simulink model "CRA_Assignment2"  (R2022b)
settings: Solver=ode23  StartTime=0.0  StopTime=10  RelTol=1e-7  AbsTol=1e-7
libraries: simulink x2
settings Model: Creator=gianm  LastModifiedBy=lerio

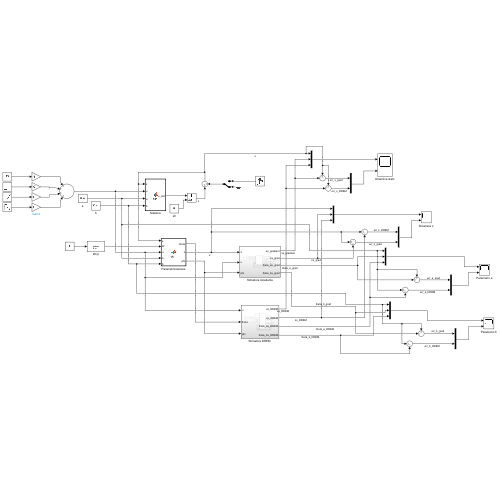
[thumbnail: Simulink's stored preview of the top-level diagram]
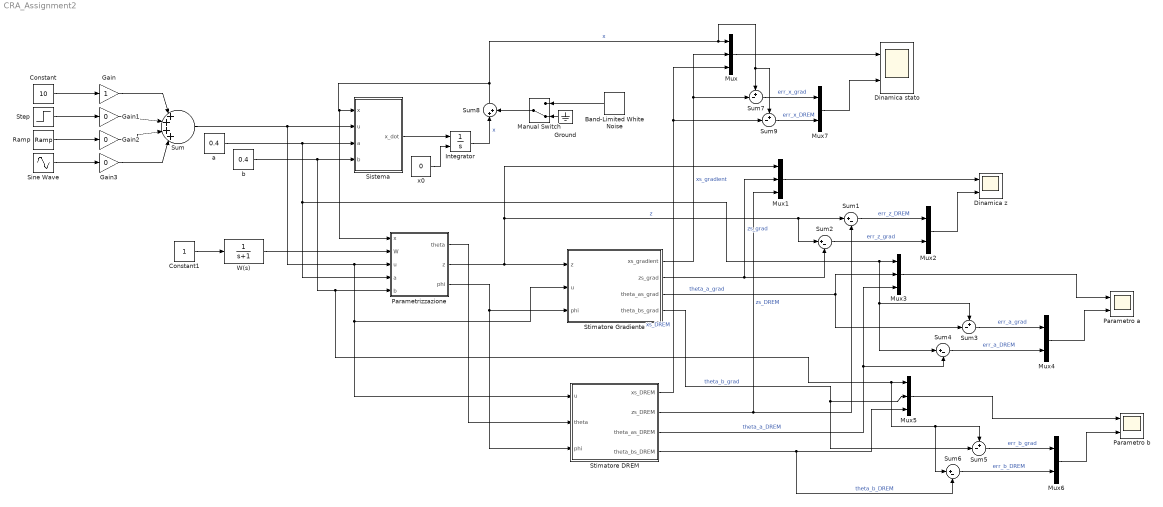
== system CRA_Assignment2 ==
  Band-Limited White Noise : simulink/Sources/Band-Limited White Noise  Cov=[0.02]  Ts=0.1  seed=[23341]
  Constant : Constant  Value=10
  Constant1 : Constant
  Dinamica stato : Scope  NumInputPorts=2
  Dinamica z : Scope  NumInputPorts=2
  Gain : Gain
  Gain1 : Gain  Gain=0
  Gain2 : Gain  Gain=0
  Gain3 : Gain  Gain=0
  Ground : Ground
  Integrator : Integrator  InitialConditionSource=external
  Manual Switch : ManualSwitch  CurrentSetting=0
  Mux{,1,3,5} (4 alike) : Mux  Inputs=3
  Mux{2,4,6..7} (4 alike) : Mux  Inputs=2
  Parametrizzazione : MATLAB Function  TreatAsAtomicUnit=on
  Parametro a : Scope  NumInputPorts=2
  Parametro b : Scope  NumInputPorts=2
  Ramp : simulink/Sources/Ramp  slope=1  start=0  InitialOutput=0
  Sine Wave : Sin  Amplitude=10  Frequency=5/2  SampleTime=0
  Sistema : MATLAB Function  TreatAsAtomicUnit=on
  Step : Step  After=10  SampleTime=0
  "Stimatore DREM " : Subsystem
  Stimatore Gradiente : Subsystem
  Sum : Sum  Inputs=|++++|
  Sum{1..2,4,6} (4 alike) : Sum  Inputs=|+-
  Sum{3,5,7,9} (4 alike) : Sum  Inputs=+-|
  Sum8 : Sum  Inputs=|++
  W(s) : TransferFcn  Denominator=[1 1]
  a : Constant  Value=0.4
  b : Constant  Value=0.4
  x0 : Constant  Value=0
  wires:
  Sistema/1(x_dot) -> Integrator/1
  Gain/1 -> Sum/1
  Gain1/1 -> Sum/2
  Gain2/1 -> Sum/3
  Gain3/1 -> Sum/4
  Sum/1 -> "Stimatore DREM "/1(u), Stimatore Gradiente/2(u), Parametrizzazione/3(u), Sistema/2(u)
  Constant/1 -> Gain/1
  Step/1 -> Gain1/1
  Ramp/1 -> Gain2/1
  Sine Wave/1 -> Gain3/1
  b/1 -> Sum6/1, Sum5/1, Mux5/1, Parametrizzazione/5(b), Sistema/4(b)
  a/1 -> Sum3/1, Sum4/1, Mux3/1, Parametrizzazione/4(a), Sistema/3(a)
  Constant1/1 -> W(s)/1
  W(s)/1 -> Parametrizzazione/2(W)
  Parametrizzazione/3(phi) -> "Stimatore DREM "/3(phi), Stimatore Gradiente/3(phi)
  Parametrizzazione/2(z) -> Sum2/1, Sum1/1, Mux1/1, Stimatore Gradiente/1(z)  "z"
  Parametrizzazione/1(theta) -> "Stimatore DREM "/2(theta)
  x0/1 -> Integrator/2
  Mux/1 -> Dinamica stato/1
  Stimatore Gradiente/1(xs_gradient) -> Sum7/2, Mux/2  "xs_gradient"
  "Stimatore DREM "/1(xs_DREM) -> Sum9/2, Mux/3  "xs_DREM"
  Stimatore Gradiente/2(zs_grad) -> Sum2/2, Mux1/2  "zs_grad"
  "Stimatore DREM "/2(zs_DREM) -> Sum1/2, Mux1/3  "zs_DREM"
  Mux1/1 -> Dinamica z/1
  Sum1/1 -> Mux2/1  "err_z_DREM"
  Sum2/1 -> Mux2/2  "err_z_grad"
  Mux2/1 -> Dinamica z/2
  Mux3/1 -> Parametro a/1
  Sum4/1 -> Mux4/2  "err_a_DREM"
  Mux4/1 -> Parametro a/2
  Sum3/1 -> Mux4/1  "err_a_grad"
  Stimatore Gradiente/3(theta_as_grad) -> Sum3/2, Mux3/2  "theta_a_grad"
  "Stimatore DREM "/3(theta_as_DREM) -> Sum4/2, Mux3/3  "theta_a_DREM"
  Mux6/1 -> Parametro b/2
  Sum5/1 -> Mux6/1  "err_b_grad"
  Sum6/1 -> Mux6/2  "err_b_DREM"
  Mux5/1 -> Parametro b/1
  "Stimatore DREM "/4(theta_bs_DREM) -> Mux5/3, Sum6/2  "theta_b_DREM"
  Stimatore Gradiente/4(theta_bs_grad) -> Sum5/2, Mux5/2  "theta_b_grad"
  Sum9/1 -> Mux7/2  "err_x_DREM"
  Sum7/1 -> Mux7/1  "err_x_grad"
  Mux7/1 -> Dinamica stato/2
  Integrator/1 -> Sum8/1  "x"
  Manual Switch/1 -> Sum8/2
  Ground/1 -> Manual Switch/2
  Band-Limited White Noise/1 -> Manual Switch/1
  Sum8/1 -> Sum9/1, Sum7/1, Mux/1, Parametrizzazione/1(x), Sistema/1(x)  "x"

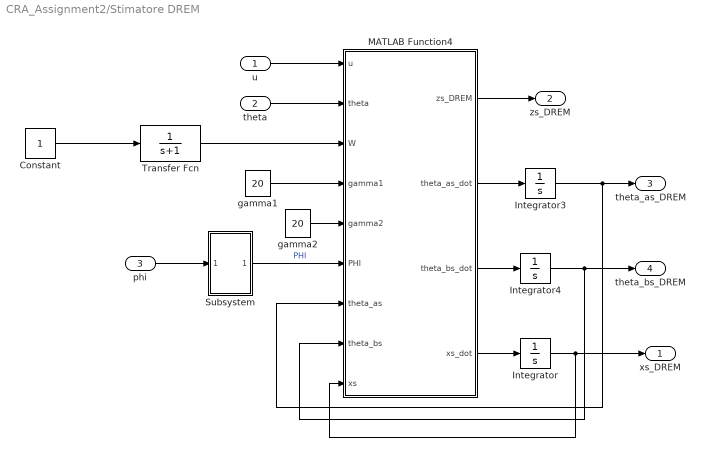
== system CRA_Assignment2/Stimatore DREM  ==
  u : Inport
  theta : Inport  Port=2
  phi : Inport  Port=3
  Constant : Constant
  Integrator : Integrator
  Integrator3 : Integrator
  Integrator4 : Integrator
  MATLAB Function4 : MATLAB Function  TreatAsAtomicUnit=on
  Subsystem : Subsystem
  Transfer Fcn : TransferFcn  Denominator=[1 1]
  gamma1 : Constant  Value=20
  gamma2 : Constant  Value=20
  xs_DREM : Outport
  zs_DREM : Outport  Port=2
  theta_as_DREM : Outport  Port=3
  theta_bs_DREM : Outport  Port=4
  wires:
  MATLAB Function4/2(theta_as_dot) -> Integrator3/1
  theta/1 -> MATLAB Function4/2(theta)
  gamma1/1 -> MATLAB Function4/4(gamma1)
  phi/1 -> Subsystem/1(phi)
  Integrator4/1 -> theta_bs_DREM/1, MATLAB Function4/8(theta_bs)
  gamma2/1 -> MATLAB Function4/5(gamma2)
  MATLAB Function4/1(zs_DREM) -> zs_DREM/1
  MATLAB Function4/3(theta_bs_dot) -> Integrator4/1
  Integrator3/1 -> MATLAB Function4/7(theta_as), theta_as_DREM/1
  Subsystem/1(PHI) -> MATLAB Function4/6(PHI)  "PHI"
  MATLAB Function4/4(xs_dot) -> Integrator/1
  Integrator/1 -> MATLAB Function4/9(xs), xs_DREM/1
  u/1 -> MATLAB Function4/1(u)
  Transfer Fcn/1 -> MATLAB Function4/3(W)
  Constant/1 -> Transfer Fcn/1

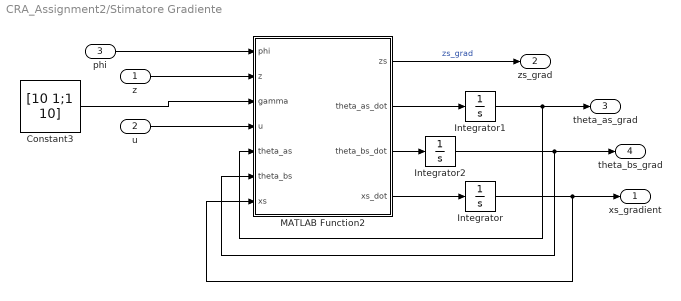
== system CRA_Assignment2/Stimatore Gradiente ==
  z : Inport
  u : Inport  Port=2
  phi : Inport  Port=3
  Constant3 : Constant  Value=[10 1;1 10]  VectorParams1D=off
  Integrator : Integrator
  Integrator1 : Integrator
  Integrator2 : Integrator
  MATLAB Function2 : MATLAB Function  TreatAsAtomicUnit=on
  xs_gradient : Outport
  zs_grad : Outport  Port=2
  theta_as_grad : Outport  Port=3
  theta_bs_grad : Outport  Port=4
  wires:
  z/1 -> MATLAB Function2/2(z)
  Integrator2/1 -> theta_bs_grad/1, MATLAB Function2/6(theta_bs)
  MATLAB Function2/3(theta_bs_dot) -> Integrator2/1
  Constant3/1 -> MATLAB Function2/3(gamma)
  Integrator1/1 -> theta_as_grad/1, MATLAB Function2/5(theta_as)
  MATLAB Function2/2(theta_as_dot) -> Integrator1/1
  phi/1 -> MATLAB Function2/1(phi)
  MATLAB Function2/1(zs) -> zs_grad/1  "zs_grad"
  MATLAB Function2/4(xs_dot) -> Integrator/1
  Integrator/1 -> xs_gradient/1, MATLAB Function2/7(xs)
  u/1 -> MATLAB Function2/4(u)

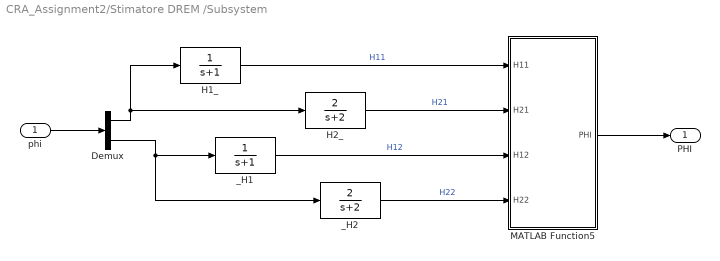
== system CRA_Assignment2/Stimatore DREM /Subsystem ==
  phi : Inport
  Demux : Demux  Outputs=2
  H1_ : TransferFcn  Denominator=[1 1]
  H2_ : TransferFcn  Numerator=[2]  Denominator=[1 2]
  MATLAB Function5 : MATLAB Function  TreatAsAtomicUnit=on
  _H1 : TransferFcn  Denominator=[1 1]
  _H2 : TransferFcn  Numerator=[2]  Denominator=[1 2]
  PHI : Outport
  wires:
  MATLAB Function5/1(PHI) -> PHI/1
  _H2/1 -> MATLAB Function5/4(H22)  "H22"
  H2_/1 -> MATLAB Function5/2(H21)  "H21"
  Demux/1 -> H2_/1, H1_/1
  Demux/2 -> _H2/1, _H1/1
  H1_/1 -> MATLAB Function5/1(H11)  "H11"
  _H1/1 -> MATLAB Function5/3(H12)  "H12"
  phi/1 -> Demux/1

== matlab function CRA_Assignment2/Parametrizzazione ==
  data: x input; W input; u input; a input; b input; theta output; z output; phi output
function [theta,z,phi]  = fcn(x,W, u,a,b)
psi = [-x;u];

theta = [a,b];
phi = W*psi;
z = theta*phi;

== matlab function CRA_Assignment2/Sistema ==
  data: x input; u input; a input; b input; x_dot output
function x_dot = fcn(x,u,a,b)

x_dot = -a*x+b*u;

== matlab function CRA_Assignment2/Stimatore Gradiente/MATLAB Function2 ==
  data: phi input; z input; zs output; gamma input; u input; theta_as_dot output; theta_bs_dot output; theta_as input; theta_bs input; xs input; xs_dot output
function [zs, theta_as_dot, theta_bs_dot, xs_dot] = fcn(phi, z, gamma, u, theta_as, theta_bs, xs)

zs = [theta_as, theta_bs]*phi;

theta_s_dot =gamma*(z-zs)*phi;
theta_as_dot = theta_s_dot(1);
theta_bs_dot = theta_s_dot(2);

xs_dot = -theta_as*xs+(theta_bs)*u;

== matlab function CRA_Assignment2/Stimatore DREM /MATLAB Function4 ==
  data: u input; zs_DREM output; theta input; W input; gamma1 input; gamma2 input; PHI input; theta_as_dot output; theta_bs_dot output; theta_as input; theta_bs input; xs input; xs_dot output
function [zs_DREM, theta_as_dot,theta_bs_dot, xs_dot] = fcn(u, theta, W, gamma1, gamma2, PHI, theta_as, theta_bs, xs)

Zs_1 = det(PHI)*theta(1);
Zs_2 = det(PHI)*theta(2);

theta_as_dot = gamma1*det(PHI)*(Zs_1-det(PHI)*theta_as);
theta_bs_dot = gamma2*det(PHI)*(Zs_2-det(PHI)*theta_bs);

theta_s = [theta_as theta_bs];
zs_DREM = W * theta_s * [-xs; u];
xs_dot = - theta_as*xs + theta_bs*u;

== matlab function CRA_Assignment2/Stimatore DREM /Subsystem/MATLAB Function5 ==
  data: H11 input; H21 input; PHI output; H12 input; H22 input
function PHI = fcn(H11, H21, H12, H22)

PHI = [H11,H12;H21,H22];
